simulink model "BiomT1_WITHPROP_Model"  (R2023b)
settings: Solver=VariableStepAuto  StartTime=0.0  StopTime=100.0  RelTol=1e-3
values from neighbouring files (symbols this model uses):
  g = num2str(Outeron_Values(outeron))    [GetCoeff_WITHPROP.m]    (also in initialize_model.m = 9.81)
  inertiaGeom = load_inertiaGeom()    [computeAeroFM.m]    (also in initialize_model.m)
  Power_Values = load("Propeller_Data1.mat", "Power_Values")    [initialize_model.m]
  RPM_Values = load("Propeller_Data1.mat", "RPM_Values")    [initialize_model.m]
  Thrust_Values = load("Propeller_Data1.mat", "Thrust_Values")    [initialize_model.m]
  x0 = [0 0 zbar u0 v0 w0 0 0 0 0 0 0]    [initialize_model.m]
libraries: simulink x4, aerolibasang x2, shared6dof x1, aerolibatmos2 x1
settings Model: Creator=sherpa  LastModifiedBy=sudip
settings SolverCC: AlgebraicLoopSolver=TrustRegion
settings OptimizationCC: ReuseModelBlockBuffer=off
settings DebuggingCC: UnconnectedInputMsg=warning  UnconnectedOutputMsg=warning  UnconnectedLineMsg=warning
settings ModelReferenceCC: EnableRefExpFcnMdlSchedulingChecks=on
settings RTWCC: DLArmComputeVersion=19.05

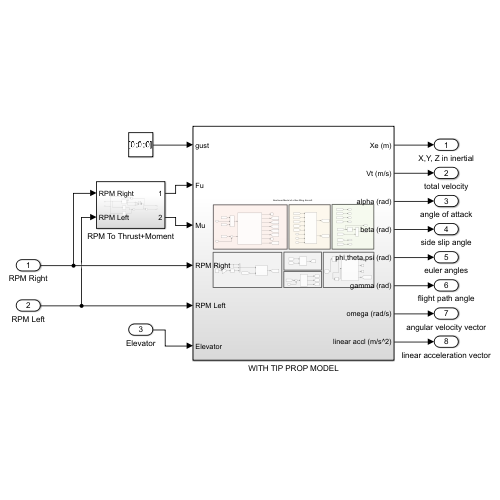
[thumbnail: Simulink's stored preview of the top-level diagram]
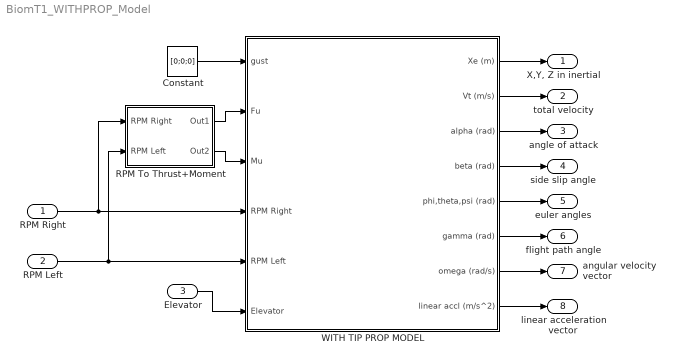
== system BiomT1_WITHPROP_Model ==
  RPM Right : Inport
  RPM Left : Inport  Port=2
  Elevator : Inport  Port=3
  Constant : Constant  Value=[0;0;0]
  RPM To Thrust+Moment : Subsystem
  WITH TIP PROP MODEL : Subsystem
  "X,Y, Z in inertial" : Outport
  total velocity : Outport  Port=2
  angle of attack : Outport  Port=3
  side slip angle : Outport  Port=4
  euler angles : Outport  Port=5
  flight path angle : Outport  Port=6
  angular velocity vector : Outport  Port=7
  linear acceleration vector : Outport  Port=8
  wires:
  WITH TIP PROP MODEL/1(Xe (m)) -> "X,Y, Z in inertial"/1
  WITH TIP PROP MODEL/2(Vt (m/s)) -> total velocity/1
  WITH TIP PROP MODEL/3(alpha (rad)) -> angle of attack/1
  WITH TIP PROP MODEL/4(beta (rad)) -> side slip angle/1
  WITH TIP PROP MODEL/6(gamma (rad)) -> flight path angle/1
  WITH TIP PROP MODEL/7(omega (rad/s)) -> angular velocity vector/1
  WITH TIP PROP MODEL/8(linear accl (m/s^2)) -> linear acceleration vector/1
  WITH TIP PROP MODEL/5(phi,theta,psi (rad)) -> euler angles/1
  Constant/1 -> WITH TIP PROP MODEL/1(gust)
  Elevator/1 -> WITH TIP PROP MODEL/6("Elevator ")
  RPM Left/1 -> WITH TIP PROP MODEL/5(RPM Left), RPM To Thrust+Moment/2(RPM Left)
  RPM To Thrust+Moment/1(Out1) -> WITH TIP PROP MODEL/2(Fu)
  RPM To Thrust+Moment/2(Out2) -> WITH TIP PROP MODEL/3(Mu)
  RPM Right/1 -> RPM To Thrust+Moment/1(RPM Right), WITH TIP PROP MODEL/4(RPM Right)

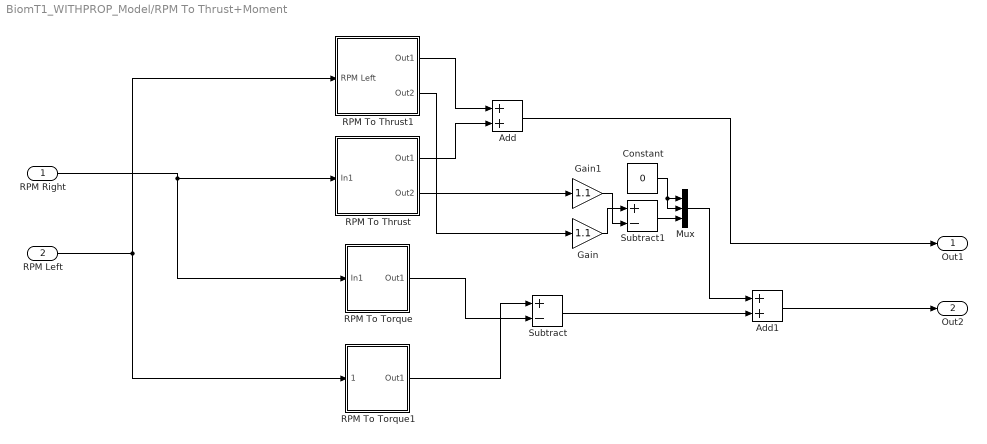
== system BiomT1_WITHPROP_Model/RPM To Thrust+Moment ==
  RPM Right : Inport
  RPM Left : Inport  Port=2
  Add : Sum
  Add1 : Sum
  Constant : Constant  Value=0
  Gain : Gain  Gain=1.1
  Gain1 : Gain  Gain=1.1
  Mux : Mux  Inputs=3
  RPM To Thrust : Subsystem
  RPM To Thrust1 : Subsystem
  RPM To Torque : Subsystem
  RPM To Torque1 : Subsystem
  Subtract : Sum  Inputs=+-
  Subtract1 : Sum  Inputs=+-
  Out1 : Outport
  Out2 : Outport  Port=2
  wires:
  RPM To Thrust/1(Out1) -> Add/2
  RPM Left/1 -> RPM To Torque1/1(RPM Left), RPM To Thrust1/1(RPM Left)
  RPM To Thrust1/1(Out1) -> Add/1
  RPM To Torque/1(Out1) -> Subtract/2
  RPM Right/1 -> RPM To Torque/1(In1), RPM To Thrust/1(In1)
  RPM To Torque1/1(Out1) -> Subtract/1
  Add/1 -> Out1/1
  RPM To Thrust1/2(Out2) -> Gain/1
  RPM To Thrust/2(Out2) -> Gain1/1
  Subtract1/1 -> Mux/3
  Constant/1 -> Mux/1, Mux/2
  Mux/1 -> Add1/1
  Subtract/1 -> Add1/2
  Add1/1 -> Out2/1
  Gain1/1 -> Subtract1/2
  Gain/1 -> Subtract1/1

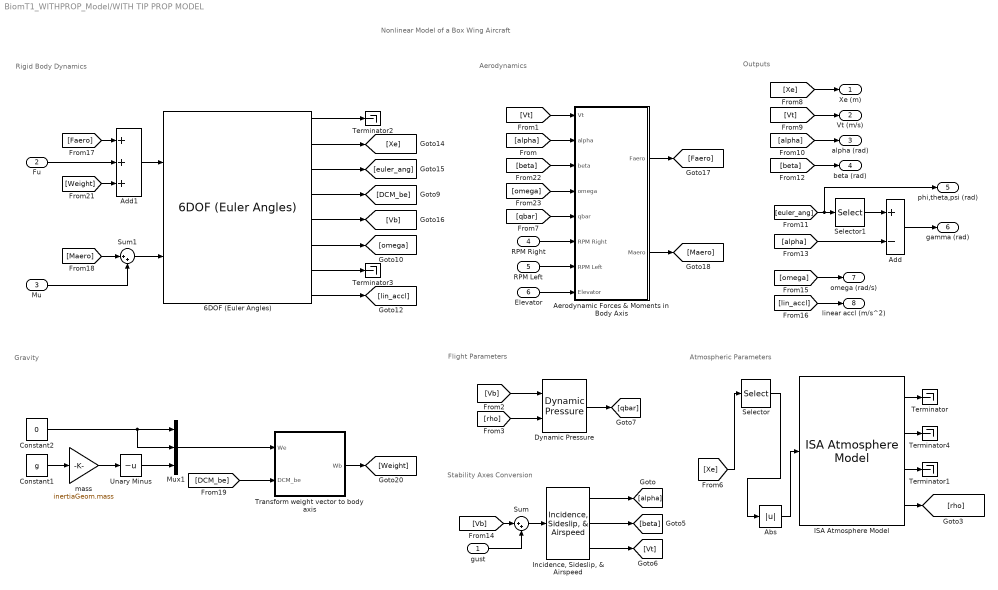
== system BiomT1_WITHPROP_Model/WITH TIP PROP MODEL ==
  note: Gravity
  note: Nonlinear Model of a Box Wing Aircraft
  note: Aerodynamics
  note: Outputs
  note: Rigid Body Dynamics
  note: Stability Axes Conversion
  note: Atmospheric Parameters
  note: Flight Parameters
  gust : Inport  PortDimensions=3
  Fu : Inport  Port=2  PortDimensions=3
  Mu : Inport  Port=3  PortDimensions=3
  RPM Right : Inport  Port=4
  RPM Left : Inport  Port=5
  "Elevator " : Inport  Port=6
  6DOF (Euler Angles) : shared6dof/6DOF (Euler Angles)  units=Metric (MKS)  mtype=Fixed  rep=Euler Angles  xme_0=x0(1:3)  Vm_0=x0(4:6)  eul_0=x0(7:9)  pm_0=x0(10:12)  mass_0=inertiaGeom.mass  mass_e=0.5  mass_f=2.0  inertia=inertiaGeom.inertiaMatrix  inertia_e=eye(3)  inertia_f=2*eye(3)  k_quat=1.0  vre_flag=on  abi_flag=off  aMode=0  xme_statename={'Xe','Ye','Ze'}  Vm_statename={'U','v','w'}  eul_statename={'phi','theta','psi'}  quat_statename=''  pm_statename={'p','q','r'}  mass_statename=''
  Abs : Abs  SaturateOnIntegerOverflow=off
  Add : Sum  Inputs=+-
  Add1 : Sum  Inputs=+++
  Aerodynamic Forces & Moments in Body Axis : Subsystem
  Constant1 : Constant  Value=g
  Constant2 : Constant  Value=0
  Dynamic Pressure : aerolibasang/Dynamic Pressure
  ISA Atmosphere Model : aerolibatmos2/ISA Atmosphere Model  useExtended=off  action=Warning  custom=off  viscosityOut=off  g=9.80665  gamma=1.4  R=287.0531  L=0.0065  h_trop=11000  h_strat=20000  rho0=1.225  P0=101325  T0=288.15  h0=0
  "Incidence, Sideslip, & Airspeed" : aerolibasang/Incidence, Sideslip, & Airspeed
  Mux1 : Mux  Inputs=3
  Selector : Selector  InputPortWidth=3  IndexOptions=Index vector (dialog)  Indices=3  OutputSizes=1
  Selector1 : Selector  InputPortWidth=3  IndexOptions=Index vector (dialog)  Indices=2  OutputSizes=1
  Sum : Sum  Inputs=|++
  Sum1 : Sum  Inputs=|++
  Terminator{,1..4} (5 alike) : Terminator
  Transform weight vector to body axis : MATLAB Function  TreatAsAtomicUnit=on
  Unary Minus : UnaryMinus
  mass : Gain  Gain=inertiaGeom.mass
  Xe (m) : Outport
  Vt (m/s) : Outport  Port=2
  alpha (rad) : Outport  Port=3
  beta (rad) : Outport  Port=4
  phi,theta,psi (rad) : Outport  Port=5
  gamma (rad) : Outport  Port=6
  omega (rad/s) : Outport  Port=7
  linear accl (m/s^2) : Outport  Port=8
  wires:
  [Xe] -> Selector/1
  [beta] -> beta (rad)/1
  "Incidence, Sideslip, & Airspeed"/3 -> [Vt]
  ISA Atmosphere Model/3 -> Terminator1/1
  ISA Atmosphere Model/1 -> Terminator/1
  ISA Atmosphere Model/4 -> [rho]
  [rho] -> Dynamic Pressure/2
  6DOF (Euler Angles)/3 -> [euler_ang]
  [lin_accl] -> linear accl (m/s^2)/1
  [alpha] -> alpha (rad)/1
  ISA Atmosphere Model/2 -> Terminator4/1
  [Vb] -> Dynamic Pressure/1
  6DOF (Euler Angles)/2 -> [Xe]
  Add/1 -> gamma (rad)/1
  [Vt] -> Vt (m/s)/1
  6DOF (Euler Angles)/7 -> Terminator3/1
  "Incidence, Sideslip, & Airspeed"/2 -> [beta]
  Selector1/1 -> Add/1
  6DOF (Euler Angles)/8 -> [lin_accl]
  6DOF (Euler Angles)/1 -> Terminator2/1
  6DOF (Euler Angles)/6 -> [omega]
  6DOF (Euler Angles)/4 -> [DCM_be]
  "Incidence, Sideslip, & Airspeed"/1 -> [alpha]
  [alpha] -> Add/2
  6DOF (Euler Angles)/5 -> [Vb]
  [euler_ang] -> phi,theta,psi (rad)/1, Selector1/1
  [omega] -> omega (rad/s)/1
  Dynamic Pressure/1 -> [qbar]
  [Xe] -> Xe (m)/1
  Constant1/1 -> mass/1
  mass/1 -> Unary Minus/1
  Unary Minus/1 -> Mux1/3
  Mux1/1 -> Transform weight vector to body axis/1(We)
  Transform weight vector to body axis/1(Wb) -> [Weight]
  [DCM_be] -> Transform weight vector to body axis/2(DCM_be)
  Constant2/1 -> Mux1/2, Mux1/1
  [Faero] -> Add1/1
  Fu/1 -> Add1/2
  [Weight] -> Add1/3
  Add1/1 -> 6DOF (Euler Angles)/1
  [alpha] -> Aerodynamic Forces & Moments in Body Axis/2(alpha)
  [qbar] -> Aerodynamic Forces & Moments in Body Axis/5(qbar)
  Aerodynamic Forces & Moments in Body Axis/1(Faero) -> [Faero]
  Aerodynamic Forces & Moments in Body Axis/2(Maero) -> [Maero]
  [omega] -> Aerodynamic Forces & Moments in Body Axis/4(omega)
  [beta] -> Aerodynamic Forces & Moments in Body Axis/3(beta)
  [Vt] -> Aerodynamic Forces & Moments in Body Axis/1(Vt)
  [Vb] -> Sum/1
  Sum/1 -> "Incidence, Sideslip, & Airspeed"/1
  gust/1 -> Sum/2
  Sum1/1 -> 6DOF (Euler Angles)/2
  [Maero] -> Sum1/1
  Mu/1 -> Sum1/2
  "Elevator "/1 -> Aerodynamic Forces & Moments in Body Axis/8("Elevator ")
  Selector/1 -> Abs/1
  Abs/1 -> ISA Atmosphere Model/1
  RPM Right/1 -> Aerodynamic Forces & Moments in Body Axis/6(RPM Right)
  RPM Left/1 -> Aerodynamic Forces & Moments in Body Axis/7(RPM Left)

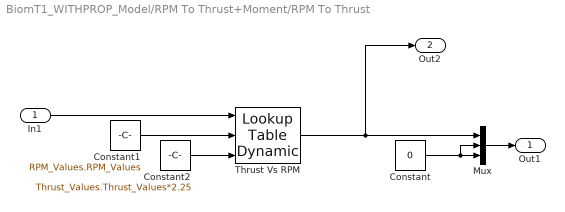
== system BiomT1_WITHPROP_Model/RPM To Thrust+Moment/RPM To Thrust ==
  In1 : Inport
  Constant : Constant  Value=0
  Constant1 : Constant  Value=RPM_Values.RPM_Values
  Constant2 : Constant  Value=Thrust_Values.Thrust_Values*2.25
  Mux : Mux  Inputs=3
  Thrust Vs RPM : simulink/Lookup Tables/Lookup Table Dynamic  LookUpMeth=Interpolation-Use End Values  OutDataType=fixdt('double')  OutScaling=[]  OutputDataTypeScalingMode=Specify via dialog  OutDataTypeStr=double  DoSatur=off
  Out1 : Outport
  Out2 : Outport  Port=2
  wires:
  Constant2/1 -> Thrust Vs RPM/3
  Constant1/1 -> Thrust Vs RPM/2
  In1/1 -> Thrust Vs RPM/1
  Constant/1 -> Mux/3, Mux/2
  Mux/1 -> Out1/1
  Thrust Vs RPM/1 -> Out2/1, Mux/1

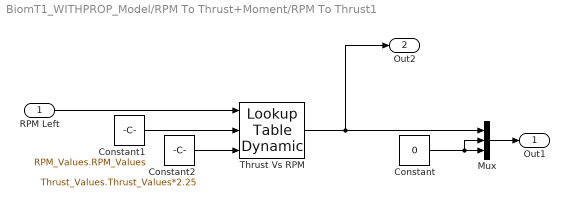
== system BiomT1_WITHPROP_Model/RPM To Thrust+Moment/RPM To Thrust1 ==
  RPM Left : Inport
  Constant : Constant  Value=0
  Constant1 : Constant  Value=RPM_Values.RPM_Values
  Constant2 : Constant  Value=Thrust_Values.Thrust_Values*2.25
  Mux : Mux  Inputs=3
  Thrust Vs RPM : simulink/Lookup Tables/Lookup Table Dynamic  LookUpMeth=Interpolation-Use End Values  OutDataType=fixdt('double')  OutScaling=[]  OutputDataTypeScalingMode=Specify via dialog  OutDataTypeStr=double  DoSatur=off
  Out1 : Outport
  Out2 : Outport  Port=2
  wires:
  Mux/1 -> Out1/1
  Thrust Vs RPM/1 -> Out2/1, Mux/1
  Constant/1 -> Mux/2, Mux/3
  RPM Left/1 -> Thrust Vs RPM/1
  Constant1/1 -> Thrust Vs RPM/2
  Constant2/1 -> Thrust Vs RPM/3

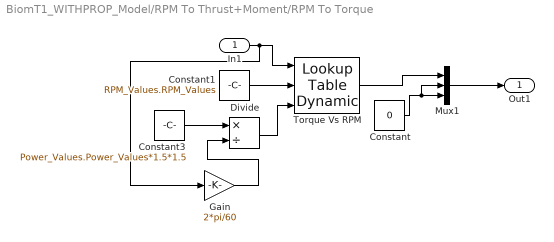
== system BiomT1_WITHPROP_Model/RPM To Thrust+Moment/RPM To Torque ==
  In1 : Inport
  Constant : Constant  Value=0
  Constant1 : Constant  Value=RPM_Values.RPM_Values
  Constant3 : Constant  Value=Power_Values.Power_Values*1.5*1.5
  Divide : Product  Inputs=*/
  Gain : Gain  Gain=2*pi/60
  Mux1 : Mux  Inputs=3
  Torque Vs RPM : simulink/Lookup Tables/Lookup Table Dynamic  LookUpMeth=Interpolation-Use End Values  OutDataType=fixdt('double')  OutScaling=[]  OutputDataTypeScalingMode=Specify via dialog  OutDataTypeStr=double  DoSatur=off
  Out1 : Outport
  wires:
  In1/1 -> Gain/1, Torque Vs RPM/1
  Constant1/1 -> Torque Vs RPM/2
  Constant/1 -> Mux1/2, Mux1/3
  Mux1/1 -> Out1/1
  Constant3/1 -> Divide/1
  Divide/1 -> Torque Vs RPM/3
  Gain/1 -> Divide/2
  Torque Vs RPM/1 -> Mux1/1

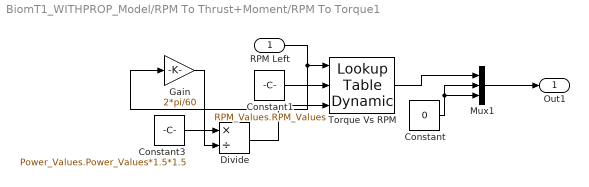
== system BiomT1_WITHPROP_Model/RPM To Thrust+Moment/RPM To Torque1 ==
  RPM Left : Inport
  Constant : Constant  Value=0
  Constant1 : Constant  Value=RPM_Values.RPM_Values
  Constant3 : Constant  Value=Power_Values.Power_Values*1.5*1.5
  Divide : Product  Inputs=*/
  Gain : Gain  Gain=2*pi/60
  Mux1 : Mux  Inputs=3
  Torque Vs RPM : simulink/Lookup Tables/Lookup Table Dynamic  LookUpMeth=Interpolation-Use End Values  OutDataType=fixdt('double')  OutScaling=[]  OutputDataTypeScalingMode=Specify via dialog  OutDataTypeStr=double  DoSatur=off
  Out1 : Outport
  wires:
  Mux1/1 -> Out1/1
  Constant/1 -> Mux1/2, Mux1/3
  Torque Vs RPM/1 -> Mux1/1
  Constant1/1 -> Torque Vs RPM/2
  RPM Left/1 -> Gain/1, Torque Vs RPM/1
  Constant3/1 -> Divide/1
  Divide/1 -> Torque Vs RPM/3
  Gain/1 -> Divide/2

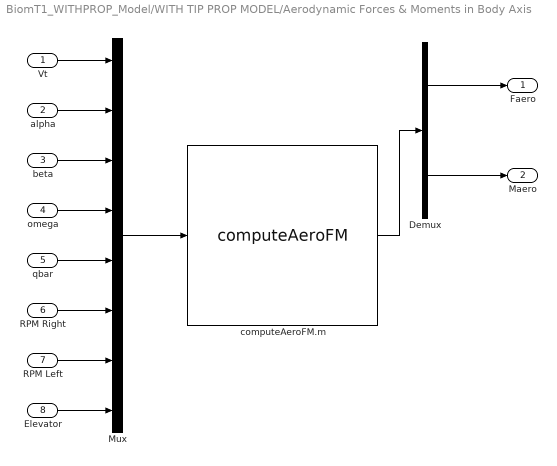
== system BiomT1_WITHPROP_Model/WITH TIP PROP MODEL/Aerodynamic Forces & Moments in Body Axis ==
  Vt : Inport
  alpha : Inport  Port=2
  beta : Inport  Port=3
  omega : Inport  Port=4
  qbar : Inport  Port=5
  RPM Right : Inport  Port=6
  RPM Left : Inport  Port=7
  "Elevator " : Inport  Port=8
  Demux : Demux  Outputs=2
  Mux : Mux  Inputs=8
  computeAeroFM.m : MATLABFcn  MATLABFcn=computeAeroFM  OutputDimensions=6  OutputSignalType=real
  Faero : Outport  PortDimensions=3
  Maero : Outport  Port=2  PortDimensions=3
  wires:
  Mux/1 -> computeAeroFM.m/1
  computeAeroFM.m/1 -> Demux/1
  Demux/1 -> Faero/1
  Demux/2 -> Maero/1
  qbar/1 -> Mux/5
  Vt/1 -> Mux/1
  omega/1 -> Mux/4
  beta/1 -> Mux/3
  alpha/1 -> Mux/2
  RPM Right/1 -> Mux/6
  RPM Left/1 -> Mux/7
  "Elevator "/1 -> Mux/8

== matlab function BiomT1_WITHPROP_Model/WITH TIP PROP MODEL/Transform weight vector to body axis ==
  data: We input; Wb output; DCM_be input
function Wb = fcn(We,DCM_be)
Wb = DCM_be'*We; % Weight in body coordinate system.
